simulink library "MESSIN_Library"  (R2024a)
settings: Solver=VariableStepAuto  StartTime=0.0  StopTime=10.0  RelTol=1e-3
undefined symbols (not defined in the file or in its folder): actuatorCommand, commandedActuator, commandMode, externCommand, ready, remoteControlDevice, sensor, supervisor, timestampUTC, useXNAllocation
libraries: $bdroot x376, etargetslib x52, simulink x19
(part 1 of 5)
settings Model: Creator=damerius  LastModifiedBy=Scythe
settings OptimizationCC: ReuseModelBlockBuffer=off
settings RTWCC: GPUComputeCapability=3.5

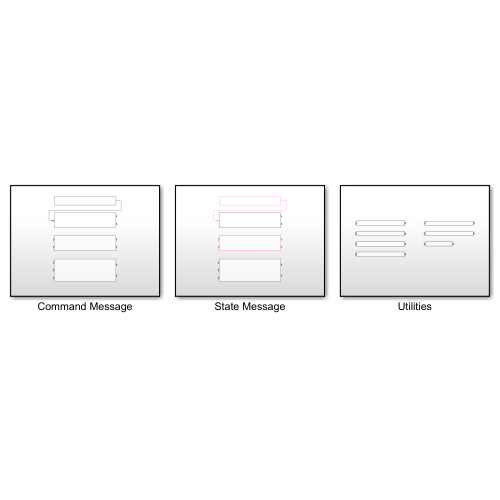
[thumbnail: Simulink's stored preview of the top-level diagram]
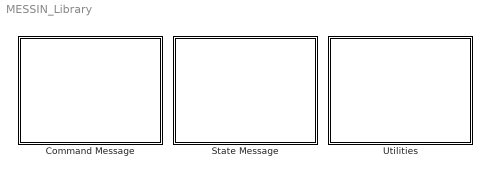
== system MESSIN_Library ==
  Command Message : Subsystem
  State Message : Subsystem
  Utilities : Subsystem

== system MESSIN_Library/Command Message ==
  Empty MESSIN Command Bus : Subsystem
      mask help: Construct an empty MESSIN command bus with default values.
      mask DialogControl DescGroupVar Prompt: Empty MESSIN Command Bus
      mask Display:
      | text(0.05, 0.5, '{\bfEmpty Bus}','horizontalAlignment','left','verticalAlignment','bottom','texmode','on');
      | text(0.05, 0.5, 'messinCommand','horizontalAlignment','left','verticalAlignment','top');
  Pack MESSIN Command Message : Subsystem
      mask help: Pack a MESSIN command message from the MESSIN command bus.
      mask DialogControl DescGroupVar Prompt: Pack MESSIN Command Message
      mask Display:
      | text(0.5, 0.5, '{\bfPack Message}','horizontalAlignment','center','verticalAlignment','bottom','texmode','on');
      | text(0.5, 0.5, 'MESSIN Command Message','horizontalAlignment','center','verticalAlignment','top');
  Unpack All MESSIN Command Messages : Subsystem
      mask help: Unpack all MESSIN command messages and construct a MESSIN command bus. If unpacking failed, then the success output returns false.
      mask DialogControl DescGroupVar Prompt: Unpack All MESSIN Command Messages
      mask Display:
      | text(0.5, 0.5, '{\bfUnpack All Messages}','horizontalAlignment','center','verticalAlignment','bottom','texmode','on');
      | text(0.5, 0.5, 'MESSIN Command Message','horizontalAlignment','center','verticalAlignment','top');
  Unpack MESSIN Command Message : Subsystem
      mask help: Unpack a MESSIN command message and construct a MESSIN command bus. If unpacking failed, then the success output returns false.
      mask DialogControl DescGroupVar Prompt: Unpack MESSIN Command Message
      mask Display:
      | text(0.5, 0.5, '{\bfUnpack Message}','horizontalAlignment','center','verticalAlignment','bottom','texmode','on');
      | text(0.5, 0.5, 'MESSIN Command Message','horizontalAlignment','center','verticalAlignment','top');
  wires:
  Empty MESSIN Command Bus/1(messinCommand) -> Pack MESSIN Command Message/1(messinCommand)

== system MESSIN_Library/State Message ==
  Empty MESSIN State Bus : Subsystem
      mask help: Construct an empty MESSIN state bus with default values.
      mask DialogControl DescGroupVar Prompt: Empty MESSIN State Bus
      mask Display:
      | text(0.05, 0.5, '{\bfEmpty Bus}','horizontalAlignment','left','verticalAlignment','bottom','texmode','on');
      | text(0.05, 0.5, 'messinState','horizontalAlignment','left','verticalAlignment','top');
  Pack MESSIN State Message : Subsystem
      mask help: Pack a MESSIN state message from the MESSIN state bus.
      mask DialogControl DescGroupVar Prompt: Pack MESSIN State Message
      mask Display:
      | text(0.5, 0.5, '{\bfPack Message}','horizontalAlignment','center','verticalAlignment','bottom','texmode','on');
      | text(0.5, 0.5, 'MESSIN State Message','horizontalAlignment','center','verticalAlignment','top');
  Unpack All MESSIN State Messages : Subsystem
      mask help: Unpack all MESSIN state messages and construct a MESSIN state bus. If unpacking failed, then the success output returns false.
      mask DialogControl DescGroupVar Prompt: Unpack All MESSIN State Messages
      mask Display:
      | text(0.5, 0.5, '{\bfUnpack All Messages}','horizontalAlignment','center','verticalAlignment','bottom','texmode','on');
      | text(0.5, 0.5, 'MESSIN State Message','horizontalAlignment','center','verticalAlignment','top');
  Unpack MESSIN State Message : Subsystem
      mask help: Unpack a MESSIN state message and construct a MESSIN state bus. If unpacking failed, then the success output returns false.
      mask DialogControl DescGroupVar Prompt: Unpack MESSIN State Message
      mask Display:
      | text(0.5, 0.5, '{\bfUnpack Message}','horizontalAlignment','center','verticalAlignment','bottom','texmode','on');
      | text(0.5, 0.5, 'MESSIN State Message','horizontalAlignment','center','verticalAlignment','top');
  wires:
  Empty MESSIN State Bus/1(messinState) -> Pack MESSIN State Message/1(messinState)

== system MESSIN_Library/Utilities ==
  Convert Double Network Byte Order : Subsystem
      mask DialogControl DescGroupVar Prompt: Convert Double Network Byte Order
      mask Display: disp('Network Byte Order (double)');
  Convert Single Network Byte Order : Subsystem
      mask DialogControl DescGroupVar Prompt: Convert Single Network Byte Order
      mask Display: disp('Network Byte Order (single)');
  Convert Uint16 Network Byte Order : Subsystem
      mask DialogControl DescGroupVar Prompt: Convert Uint16 Network Byte Order
      mask Display: disp('Network Byte Order (uint16)');
  Convert Uint32 Network Byte Order : Subsystem
      mask DialogControl DescGroupVar Prompt: Convert Uint32 Network Byte Order
      mask Display: disp('Network Byte Order (uint32)');
  Make Finite : Subsystem
      mask help: Make all values finite by replacing nonfinite values by zero.
      mask DialogControl DescGroupVar Prompt: Make Finite
      mask Display: disp('Make Finite');
  Pack Bitfield : Subsystem
      mask help: Convert a bitfield of 8 bits to a single byte. The input bitfield must be a vector containing 8 boolean values where the first value indicates whether the LSBit is to be set or not.
      mask DialogControl DescGroupVar Prompt: Pack Bitfield
      mask Display: disp('Pack Bitfield');
  Unpack Bitfield : Subsystem
      mask help: Extract all bits from a single byte. The bitfield output contains 8 boolean values where the first value indicates whether the LSBit is set or not.
      mask DialogControl DescGroupVar Prompt: Unpack Bitfield
      mask Display: disp('Unpack Bitfield');

== system MESSIN_Library/Command Message/Empty MESSIN Command Bus ==
  Bus Creator : BusCreator  Inputs=6
  Constant : Constant  Value=0.0  OutDataTypeStr=double
  Constant1 : Constant  Value=0  OutDataTypeStr=uint8
  Constant2 : Constant  Value=false  OutDataTypeStr=boolean
  Constant3 : Constant  Value=false  OutDataTypeStr=boolean
  Empty Actuator Command Bus : Subsystem
  Empty Allocation Command Bus : Subsystem
  Signal Specification : SignalSpecification  OutDataTypeStr=double  Unit=s  Dimensions=1
  Signal Specification1 : SignalSpecification  OutDataTypeStr=uint8  Dimensions=1
  Signal Specification2 : SignalSpecification  OutDataTypeStr=boolean  Dimensions=1
  Signal Specification3 : SignalSpecification  OutDataTypeStr=boolean  Dimensions=1
  messinCommand : Outport
  wires:
  Constant/1 -> Signal Specification/1
  Signal Specification/1 -> Bus Creator/1  "timestampUTC"
  Bus Creator/1 -> messinCommand/1
  Empty Actuator Command Bus/1(actuatorCommand) -> Bus Creator/5  "actuatorCommand"
  Empty Allocation Command Bus/1(allocationCommand) -> Bus Creator/6  "allocationCommand"
  Constant1/1 -> Signal Specification1/1
  Signal Specification1/1 -> Bus Creator/4  "commandMode"
  Constant2/1 -> Signal Specification2/1
  Signal Specification2/1 -> Bus Creator/2  "ready"
  Constant3/1 -> Signal Specification3/1
  Signal Specification3/1 -> Bus Creator/3  "useXNAllocation"

== system MESSIN_Library/Command Message/Pack MESSIN Command Message ==
  note: Info
  note: Commands
  note: Header
  messinCommand : Inport
  Bus Selector : BusSelector  OutputSignals=actuatorCommand
  Bus Selector1 : BusSelector  OutputSignals=allocationCommand
  Pack ActuatorCommand : Subsystem
  Pack AllocationCommand : Subsystem
  Pack Header : Subsystem
  Pack Info : Subsystem
  Vector Concatenate1 : Concatenate  NumInputs=4
  Width : Width  DataType=uint32
  messinCommand1 : InportShadow
  bytes : Outport  OutDataTypeStr=uint8
  length : Outport  Port=2  OutDataTypeStr=uint32  PortDimensions=1
  wires:
  messinCommand/1 -> Pack Info/1(messinCommand)
  Width/1 -> length/1
  Vector Concatenate1/1 -> Width/1, bytes/1
  messinCommand1/1 -> Bus Selector1/1, Bus Selector/1
  Bus Selector/1 -> Pack ActuatorCommand/1(actuatorCommand)  "<actuatorCommand>"
  Pack ActuatorCommand/1(bytes) -> Vector Concatenate1/3
  Pack Header/1(bytes) -> Vector Concatenate1/1
  Pack Info/1(bytes) -> Vector Concatenate1/2
  Bus Selector1/1 -> Pack AllocationCommand/1(allocationCommand)  "<allocationCommand>"
  Pack AllocationCommand/1(bytes) -> Vector Concatenate1/4

== system MESSIN_Library/Command Message/Unpack All MESSIN Command Messages ==
  note: protection for invalid input dimension
  bytes : Inport  OutDataTypeStr=uint8
  length : Inport  Port=2  OutDataTypeStr=uint32
  numMessages : Inport  Port=3  OutDataTypeStr=uint32  PortDimensions=1
  AND : Logic  Inputs=3  AllPortsSameDT=off  OutDataTypeStr=boolean
  Compare To Zero : simulink/Logic and Bit Operations/Compare To Zero  relop=>  OutDataTypeStr=boolean
  Compare To Zero1 : simulink/Logic and Bit Operations/Compare To Zero  relop=>  OutDataTypeStr=boolean
  Probe : Probe  ProbeWidth=off  ProbeSampleTime=off  ProbeComplexSignal=off  ProbeSignalDimensions=on  ProbeDimensionsDataType=uint32
  Relational Operator : RelationalOperator  Operator===  OutDataTypeStr=boolean  RndMeth=Simplest  InputSameDT=off
  Selector : Selector  InputPortWidth=2  IndexOptions=Index vector (dialog)  Indices=2  OutputSizes=1
  Sum of Elements : Sum  Inputs=+
  Width1 : Width  DataType=uint32
  run unpacking : Subsystem
  success : Outport  OutDataTypeStr=boolean  PortDimensions=1
  messinCommand : Outport  Port=2
  wires:
  run unpacking/1(messinCommand) -> messinCommand/1
  Compare To Zero1/1 -> AND/3
  run unpacking/2(vecUnpacked) -> Sum of Elements/1
  Relational Operator/1 -> AND/1, run unpacking/Enable
  Probe/1 -> Selector/1
  length/1 -> run unpacking/2(length), Width1/1
  Selector/1 -> Relational Operator/1
  bytes/1 -> Probe/1, run unpacking/1(bytes)
  numMessages/1 -> run unpacking/3(numMessages), Compare To Zero1/1
  AND/1 -> success/1
  Compare To Zero/1 -> AND/2
  Sum of Elements/1 -> Compare To Zero/1
  Width1/1 -> Relational Operator/2

== system MESSIN_Library/Command Message/Unpack MESSIN Command Message ==
  note: check length and header bytes
  bytes : Inport  OutDataTypeStr=uint8
  length : Inport  Port=2  OutDataTypeStr=uint32  PortDimensions=1
  is a valid message : Subsystem
  unpack message : Subsystem  TreatAsAtomicUnit=on
  success : Outport  OutDataTypeStr=boolean  PortDimensions=1
  messinCommand : Outport  Port=2
  wires:
  unpack message/1(messinCommand) -> messinCommand/1
  is a valid message/1(validMessage) -> success/1, unpack message/Enable
  length/1 -> is a valid message/1(length)
  bytes/1 -> is a valid message/2(bytes), unpack message/1(bytes)

== system MESSIN_Library/State Message/Empty MESSIN State Bus ==
  Bus Creator : BusCreator  Inputs=8
  Bus Creator1 : BusCreator  Inputs=6
  Bus Creator2 : BusCreator  Inputs=3
  Constant1 : Constant  Value=0.0  OutDataTypeStr=double
  Empty AirMAR Bus : Subsystem
  Empty BMS Bus : Subsystem
  Empty Commanded Actuator Bus : Subsystem
  Empty Control Bus : Subsystem
  Empty DVL Bus : Subsystem
  Empty GNSS Bus : Subsystem
  Empty Guidance Bus : Subsystem
  Empty INS Bus : Subsystem
  Empty MESSIN Command Bus : $bdroot/Command Message/Empty MESSIN Command Bus
  Empty MessinDrive Bus : Subsystem
  Empty Navigation Bus : Subsystem
  Empty RCD Bus : Subsystem
  Empty Supervisor Bus : Subsystem
  Empty System Diagnostics Bus : Subsystem
  Signal Specification : SignalSpecification  OutDataTypeStr=double  Unit=s  Dimensions=1
  messinState : Outport
  wires:
  Bus Creator/1 -> messinState/1
  Constant1/1 -> Signal Specification/1
  Bus Creator1/1 -> Bus Creator/2  "sensor"
  Empty RCD Bus/1(rcd) -> Bus Creator/3  "remoteControlDevice"
  Empty MessinDrive Bus/1(messinDrive) -> Bus Creator1/6  "messinDrive"
  Empty Control Bus/1(control) -> Bus Creator2/3  "control"
  Empty System Diagnostics Bus/1(systemDiagnostics) -> Bus Creator/7  "systemDiagnostics"
  Bus Creator2/1 -> Bus Creator/5  "gnc"
  Empty Supervisor Bus/1(supervisor) -> Bus Creator/4  "supervisor"
  Empty Guidance Bus/1(guidance) -> Bus Creator2/1  "guidance"
  Empty AirMAR Bus/1(airMAR) -> Bus Creator1/4  "airMAR"
  Empty Commanded Actuator Bus/1(commandedActuator) -> Bus Creator/6  "commandedActuator"
  Empty Navigation Bus/1(navigation) -> Bus Creator2/2  "navigation"
  Empty BMS Bus/1(batteryManagementSystem) -> Bus Creator1/5  "batteryManagementSystem"
  Empty DVL Bus/1(nortekDVL1000) -> Bus Creator1/3  "nortekDVL1000"
  Empty INS Bus/1(insLFK100) -> Bus Creator1/1  "insLFK100"
  Empty GNSS Bus/1(gnssAsteRx3) -> Bus Creator1/2  "gnssAsteRx3"
  Signal Specification/1 -> Bus Creator/1  "timestampUTC"
  Empty MESSIN Command Bus/1 -> Bus Creator/8  "externCommand"

== system MESSIN_Library/State Message/Pack MESSIN State Message ==
  note: Sensor
  note: Header
  note: Info
  note: RCD
  note: Supervisor
  note: GNC
  note: System Diagnostics
  note: Extern Command
  messinState : Inport
  Bus Selector : BusSelector  OutputSignals=sensor
  Bus Selector1 : BusSelector  OutputSignals=nortekDVL1000
  Bus Selector10 : BusSelector  OutputSignals=externCommand
  Bus Selector18 : BusSelector  OutputSignals=messinDrive
  Bus Selector19 : BusSelector  OutputSignals=remoteControlDevice
  Bus Selector2 : BusSelector  OutputSignals=insLFK100
  Bus Selector3 : BusSelector  OutputSignals=supervisor
  Bus Selector4 : BusSelector  OutputSignals=batteryManagementSystem
  Bus Selector5 : BusSelector  OutputSignals=gnc
  Bus Selector6 : BusSelector  OutputSignals=airMAR
  Bus Selector7 : BusSelector  OutputSignals=gnssAsteRx3
  Bus Selector8 : BusSelector  OutputSignals=commandedActuator
  Bus Selector9 : BusSelector  OutputSignals=systemDiagnostics
  Pack AirMAR : Subsystem
  Pack BMS : Subsystem
  Pack CommandedActuator : Subsystem
  Pack DVL : Subsystem
  Pack ExternCommand : Subsystem
  Pack GNC : Subsystem
  Pack GNSS : Subsystem
  Pack Header : Subsystem
  Pack INS : Subsystem
  Pack Info : Subsystem
  Pack MessinDrive : Subsystem
  Pack RCD : Subsystem
  Pack Supervisor : Subsystem
  Pack SystemDiagnostics : Subsystem
  Vector Concatenate1 : Concatenate  NumInputs=9
  Vector Concatenate2 : Concatenate  NumInputs=6
  Width : Width  DataType=uint32
  bytes : Outport  OutDataTypeStr=uint8
  length : Outport  Port=2  OutDataTypeStr=uint32  PortDimensions=1
  wires:
  Width/1 -> length/1
  Vector Concatenate1/1 -> bytes/1, Width/1
  Bus Selector2/1 -> Pack INS/1(insLFK100)  "<insLFK100>"
  Bus Selector/1 -> Bus Selector18/1, Bus Selector4/1, Bus Selector6/1, Bus Selector1/1, Bus Selector7/1, Bus Selector2/1  "<sensor>"
  messinState/1 -> Bus Selector10/1, Bus Selector9/1, Bus Selector8/1, Bus Selector5/1, Bus Selector3/1, Bus Selector19/1, Bus Selector/1, Pack Info/1(messinState)
  Bus Selector1/1 -> Pack DVL/1(dvl)  "<nortekDVL1000>"
  Bus Selector4/1 -> Pack BMS/1(bms)  "<batteryManagementSystem>"
  Bus Selector6/1 -> Pack AirMAR/1(airMAR)  "<airMAR>"
  Bus Selector7/1 -> Pack GNSS/1(gnss)  "<gnssAsteRx3>"
  Pack DVL/1(bytes) -> Vector Concatenate2/3
  Pack AirMAR/1(bytes) -> Vector Concatenate2/4
  Pack GNSS/1(bytes) -> Vector Concatenate2/2
  Pack BMS/1(bytes) -> Vector Concatenate2/5
  Pack INS/1(bytes) -> Vector Concatenate2/1
  Pack Header/1(bytes) -> Vector Concatenate1/1
  Pack Info/1(bytes) -> Vector Concatenate1/2
  Vector Concatenate2/1 -> Vector Concatenate1/3
  Bus Selector18/1 -> Pack MessinDrive/1(messinDrive)  "<messinDrive>"
  Pack MessinDrive/1(bytes) -> Vector Concatenate2/6
  Bus Selector19/1 -> Pack RCD/1(rcd)  "<remoteControlDevice>"
  Pack RCD/1(bytes) -> Vector Concatenate1/4
  Bus Selector3/1 -> Pack Supervisor/1(supervisor)  "<supervisor>"
  Pack Supervisor/1(bytes) -> Vector Concatenate1/5
  Bus Selector5/1 -> Pack GNC/1(gnc)  "<gnc>"
  Pack GNC/1(bytes) -> Vector Concatenate1/6
  Bus Selector8/1 -> Pack CommandedActuator/1(commandedActuator)  "<commandedActuator>"
  Pack CommandedActuator/1(bytes) -> Vector Concatenate1/7
  Bus Selector9/1 -> Pack SystemDiagnostics/1(systemDiagnostics)  "<systemDiagnostics>"
  Pack SystemDiagnostics/1(bytes) -> Vector Concatenate1/8
  Bus Selector10/1 -> Pack ExternCommand/1(externCommand)  "<externCommand>"
  Pack ExternCommand/1(bytes) -> Vector Concatenate1/9

== system MESSIN_Library/State Message/Unpack All MESSIN State Messages ==
  note: protection for invalid input dimension
  bytes : Inport  OutDataTypeStr=uint8
  length : Inport  Port=2  OutDataTypeStr=uint32
  numMessages : Inport  Port=3  OutDataTypeStr=uint32  PortDimensions=1
  AND : Logic  Inputs=3  AllPortsSameDT=off  OutDataTypeStr=boolean
  Compare To Zero : simulink/Logic and Bit Operations/Compare To Zero  relop=>  OutDataTypeStr=boolean
  Compare To Zero1 : simulink/Logic and Bit Operations/Compare To Zero  relop=>  OutDataTypeStr=boolean
  Probe : Probe  ProbeWidth=off  ProbeSampleTime=off  ProbeComplexSignal=off  ProbeSignalDimensions=on  ProbeDimensionsDataType=uint32
  Relational Operator : RelationalOperator  Operator===  OutDataTypeStr=boolean  RndMeth=Simplest  InputSameDT=off
  Selector : Selector  InputPortWidth=2  IndexOptions=Index vector (dialog)  Indices=2  OutputSizes=1
  Sum of Elements : Sum  Inputs=+
  Width1 : Width  DataType=uint32
  run unpacking : Subsystem
  success : Outport  OutDataTypeStr=boolean  PortDimensions=1
  messinState : Outport  Port=2
  wires:
  Selector/1 -> Relational Operator/1
  bytes/1 -> Probe/1, run unpacking/1(bytes)
  Sum of Elements/1 -> Compare To Zero/1
  Width1/1 -> Relational Operator/2
  Probe/1 -> Selector/1
  Compare To Zero/1 -> AND/2
  length/1 -> run unpacking/2(length), Width1/1
  AND/1 -> success/1
  run unpacking/2(vecUnpacked) -> Sum of Elements/1
  Relational Operator/1 -> AND/1, run unpacking/Enable
  numMessages/1 -> run unpacking/3(numMessages), Compare To Zero1/1
  run unpacking/1(messinState) -> messinState/1
  Compare To Zero1/1 -> AND/3

== system MESSIN_Library/State Message/Unpack MESSIN State Message ==
  note: check length and header bytes
  bytes : Inport  OutDataTypeStr=uint8
  length : Inport  Port=2  OutDataTypeStr=uint32  PortDimensions=1
  is a valid message : Subsystem
  unpack message : Subsystem  TreatAsAtomicUnit=on
  success : Outport  OutDataTypeStr=boolean  PortDimensions=1
  messinState : Outport  Port=2
  wires:
  is a valid message/1(validMessage) -> success/1, unpack message/Enable
  bytes/1 -> is a valid message/2(bytes), unpack message/1(bytes)
  unpack message/1(messinState) -> messinState/1
  length/1 -> is a valid message/1(length)

== system MESSIN_Library/Utilities/Convert Double Network Byte Order ==
  note: Check endianess of this machine
      | (only swap on little-endian-based machines)
  in : Inport  OutDataTypeStr=double  PortDimensions=1
  Byte Pack : etargetslib/Byte Pack  datatypes={'double'}  byteAlign=1
  Byte Pack1 : etargetslib/Byte Pack  datatypes={'uint16'}  byteAlign=1
  Byte Unpack : etargetslib/Byte Unpack  dimensions={[1]}  datatypes={'double'}  byteAlign=1
  Constant : Constant  Value=uint16(1)
  Selector : Selector  InputPortWidth=8  IndexOptions=Index vector (dialog)  Indices=[8 7 6 5 4 3 2 1]  OutputSizes=1
  Selector2 : Selector  InputPortWidth=2  IndexOptions=Index vector (dialog)  Indices=1  OutputSizes=1
  Switch : Switch  Criteria=u2 ~= 0  SaturateOnIntegerOverflow=off  InputSameDT=off
  out : Outport  OutDataTypeStr=double  PortDimensions=1
  wires:
  Byte Unpack/1 -> Switch/1
  Selector/1 -> Byte Unpack/1
  Constant/1 -> Byte Pack1/1
  in/1 -> Switch/3, Byte Pack/1
  Selector2/1 -> Switch/2
  Byte Pack/1 -> Selector/1
  Byte Pack1/1 -> Selector2/1
  Switch/1 -> out/1

== system MESSIN_Library/Utilities/Convert Single Network Byte Order ==
  note: Check endianess of this machine
      | (only swap on little-endian-based machines)
  in : Inport  OutDataTypeStr=single  PortDimensions=1
  Byte Pack : etargetslib/Byte Pack  datatypes={'single'}  byteAlign=1
  Byte Pack1 : etargetslib/Byte Pack  datatypes={'uint16'}  byteAlign=1
  Byte Unpack : etargetslib/Byte Unpack  dimensions={[1]}  datatypes={'single'}  byteAlign=1
  Constant : Constant  Value=uint16(1)
  Selector : Selector  InputPortWidth=4  IndexOptions=Index vector (dialog)  Indices=[4 3 2 1]  OutputSizes=1
  Selector2 : Selector  InputPortWidth=2  IndexOptions=Index vector (dialog)  Indices=1  OutputSizes=1
  Switch : Switch  Criteria=u2 ~= 0  SaturateOnIntegerOverflow=off  InputSameDT=off
  out : Outport  OutDataTypeStr=single  PortDimensions=1
  wires:
  Switch/1 -> out/1
  Byte Pack1/1 -> Selector2/1
  Byte Pack/1 -> Selector/1
  Selector2/1 -> Switch/2
  in/1 -> Byte Pack/1, Switch/3
  Constant/1 -> Byte Pack1/1
  Selector/1 -> Byte Unpack/1
  Byte Unpack/1 -> Switch/1

== system MESSIN_Library/Utilities/Convert Uint16 Network Byte Order ==
  note: Check endianess of this machine
      | (only swap on little-endian-based machines)
  in : Inport  OutDataTypeStr=uint16  PortDimensions=1
  Byte Pack : etargetslib/Byte Pack  datatypes={'uint16'}  byteAlign=1
  Byte Pack1 : etargetslib/Byte Pack  datatypes={'uint16'}  byteAlign=1
  Byte Unpack : etargetslib/Byte Unpack  dimensions={[1]}  datatypes={'uint16'}  byteAlign=1
  Constant : Constant  Value=uint16(1)
  Selector : Selector  InputPortWidth=2  IndexOptions=Index vector (dialog)  Indices=[2 1]  OutputSizes=1
  Selector2 : Selector  InputPortWidth=2  IndexOptions=Index vector (dialog)  Indices=1  OutputSizes=1
  Switch : Switch  Criteria=u2 ~= 0  SaturateOnIntegerOverflow=off  InputSameDT=off
  out : Outport  OutDataTypeStr=uint16  PortDimensions=1
  wires:
  Byte Unpack/1 -> Switch/1
  Selector/1 -> Byte Unpack/1
  Constant/1 -> Byte Pack1/1
  in/1 -> Switch/3, Byte Pack/1
  Selector2/1 -> Switch/2
  Byte Pack/1 -> Selector/1
  Byte Pack1/1 -> Selector2/1
  Switch/1 -> out/1

== system MESSIN_Library/Utilities/Convert Uint32 Network Byte Order ==
  note: Check endianess of this machine
      | (only swap on little-endian-based machines)
  in : Inport  OutDataTypeStr=uint32  PortDimensions=1
  Byte Pack : etargetslib/Byte Pack  datatypes={'uint32'}  byteAlign=1
  Byte Pack1 : etargetslib/Byte Pack  datatypes={'uint16'}  byteAlign=1
  Byte Unpack : etargetslib/Byte Unpack  dimensions={[1]}  datatypes={'uint32'}  byteAlign=1
  Constant : Constant  Value=uint16(1)
  Selector : Selector  InputPortWidth=4  IndexOptions=Index vector (dialog)  Indices=[4 3 2 1]  OutputSizes=1
  Selector2 : Selector  InputPortWidth=2  IndexOptions=Index vector (dialog)  Indices=1  OutputSizes=1
  Switch : Switch  Criteria=u2 ~= 0  SaturateOnIntegerOverflow=off  InputSameDT=off
  out : Outport  OutDataTypeStr=uint32  PortDimensions=1
  wires:
  Switch/1 -> out/1
  Byte Pack1/1 -> Selector2/1
  Byte Pack/1 -> Selector/1
  Selector2/1 -> Switch/2
  in/1 -> Byte Pack/1, Switch/3
  Constant/1 -> Byte Pack1/1
  Selector/1 -> Byte Unpack/1
  Byte Unpack/1 -> Switch/1

== system MESSIN_Library/Utilities/Make Finite ==
  in : Inport  OutDataTypeStr=double
  ReplaceNonfiniteByZeros : MATLAB Function  TreatAsAtomicUnit=on
  out : Outport  OutDataTypeStr=double
  wires:
  in/1 -> ReplaceNonfiniteByZeros/1(u)
  ReplaceNonfiniteByZeros/1(y) -> out/1

== system MESSIN_Library/Utilities/Pack Bitfield ==
  bitfield : Inport  OutDataTypeStr=boolean  PortDimensions=8
  Bitwise Operator : simulink/Logic and Bit Operations/Bitwise Operator  logicop=OR  UseBitMask=off  NumInputPorts=8  BitMask=bin2dec('11011001')  BitMaskRealWorld=Stored Integer
  Data Type Conversion : DataTypeConversion  OutDataTypeStr=uint8  SaturateOnIntegerOverflow=off  RndMeth=Floor
  Demux : Demux  Outputs=8
  Shift Arithmetic : ArithShift  BitShiftNumber=1  BitShiftDirection=Left
  Shift Arithmetic1 : ArithShift  BitShiftNumber=2  BitShiftDirection=Left
  Shift Arithmetic2 : ArithShift  BitShiftNumber=3  BitShiftDirection=Left
  Shift Arithmetic3 : ArithShift  BitShiftNumber=4  BitShiftDirection=Left
  Shift Arithmetic4 : ArithShift  BitShiftNumber=5  BitShiftDirection=Left
  Shift Arithmetic5 : ArithShift  BitShiftNumber=6  BitShiftDirection=Left
  Shift Arithmetic6 : ArithShift  BitShiftNumber=7  BitShiftDirection=Left
  byte : Outport  OutDataTypeStr=uint8  PortDimensions=1
  wires:
  Demux/8 -> Shift Arithmetic6/1
  Shift Arithmetic2/1 -> Bitwise Operator/4
  Shift Arithmetic5/1 -> Bitwise Operator/7
  Shift Arithmetic6/1 -> Bitwise Operator/8
  Shift Arithmetic4/1 -> Bitwise Operator/6
  Data Type Conversion/1 -> Demux/1
  Shift Arithmetic/1 -> Bitwise Operator/2
  Shift Arithmetic3/1 -> Bitwise Operator/5
  Demux/2 -> Shift Arithmetic/1
  Demux/7 -> Shift Arithmetic5/1
  Demux/5 -> Shift Arithmetic3/1
  Demux/4 -> Shift Arithmetic2/1
  Demux/6 -> Shift Arithmetic4/1
  Demux/3 -> Shift Arithmetic1/1
  Shift Arithmetic1/1 -> Bitwise Operator/3
  Demux/1 -> Bitwise Operator/1
  bitfield/1 -> Data Type Conversion/1
  Bitwise Operator/1 -> byte/1

== system MESSIN_Library/Utilities/Unpack Bitfield ==
  byte : Inport  OutDataTypeStr=uint8  PortDimensions=1
  Bitwise Operator : simulink/Logic and Bit Operations/Bitwise Operator  logicop=AND  UseBitMask=on  BitMask=1  BitMaskRealWorld=Stored Integer
  Bitwise Operator1 : simulink/Logic and Bit Operations/Bitwise Operator  logicop=AND  UseBitMask=on  BitMask=2  BitMaskRealWorld=Stored Integer
  Bitwise Operator2 : simulink/Logic and Bit Operations/Bitwise Operator  logicop=AND  UseBitMask=on  BitMask=4  BitMaskRealWorld=Stored Integer
  Bitwise Operator3 : simulink/Logic and Bit Operations/Bitwise Operator  logicop=AND  UseBitMask=on  BitMask=8  BitMaskRealWorld=Stored Integer
  Bitwise Operator4 : simulink/Logic and Bit Operations/Bitwise Operator  logicop=AND  UseBitMask=on  BitMask=16  BitMaskRealWorld=Stored Integer
  Bitwise Operator5 : simulink/Logic and Bit Operations/Bitwise Operator  logicop=AND  UseBitMask=on  BitMask=32  BitMaskRealWorld=Stored Integer
  Bitwise Operator6 : simulink/Logic and Bit Operations/Bitwise Operator  logicop=AND  UseBitMask=on  BitMask=64  BitMaskRealWorld=Stored Integer
  Bitwise Operator7 : simulink/Logic and Bit Operations/Bitwise Operator  logicop=AND  UseBitMask=on  BitMask=128  BitMaskRealWorld=Stored Integer
  Data Type Conversion1 : DataTypeConversion  OutDataTypeStr=boolean  SaturateOnIntegerOverflow=off  RndMeth=Floor
  Mux : Mux  Inputs=8
  bitfield : Outport  OutDataTypeStr=boolean  PortDimensions=8
  wires:
  Mux/1 -> Data Type Conversion1/1
  Bitwise Operator1/1 -> Mux/2
  byte/1 -> Bitwise Operator/1, Bitwise Operator7/1, Bitwise Operator6/1, Bitwise Operator5/1, Bitwise Operator4/1, Bitwise Operator3/1, Bitwise Operator2/1, Bitwise Operator1/1
  Bitwise Operator/1 -> Mux/1
  Bitwise Operator4/1 -> Mux/5
  Bitwise Operator3/1 -> Mux/4
  Bitwise Operator2/1 -> Mux/3
  Bitwise Operator5/1 -> Mux/6
  Bitwise Operator7/1 -> Mux/8
  Bitwise Operator6/1 -> Mux/7
  Data Type Conversion1/1 -> bitfield/1

== system MESSIN_Library/Command Message/Empty MESSIN Command Bus/Empty Actuator Command Bus ==
  Bus Creator6 : BusCreator  Inputs=4
  Constant{6..8,19} (4 alike) : Constant  Value=0.0  OutDataTypeStr=double
  Signal Specification18 : SignalSpecification  OutDataTypeStr=double  Unit=1  Dimensions=1
  Signal Specification6 : SignalSpecification  OutDataTypeStr=double  Unit=1  Dimensions=1
  Signal Specification7 : SignalSpecification  OutDataTypeStr=double  Unit=rad  Dimensions=1
  Signal Specification8 : SignalSpecification  OutDataTypeStr=double  Unit=rad  Dimensions=1
  actuatorCommand : Outport
  wires:
  Signal Specification8/1 -> Bus Creator6/4  "anglePortside"
  Bus Creator6/1 -> actuatorCommand/1
  Signal Specification18/1 -> Bus Creator6/1  "throttleStarboard"
  Constant6/1 -> Signal Specification6/1
  Constant8/1 -> Signal Specification8/1
  Signal Specification6/1 -> Bus Creator6/2  "throttlePortside"
  Signal Specification7/1 -> Bus Creator6/3  "angleStarboard"
  Constant7/1 -> Signal Specification7/1
  Constant19/1 -> Signal Specification18/1

== system MESSIN_Library/Command Message/Empty MESSIN Command Bus/Empty Allocation Command Bus ==
  Bus Creator : BusCreator  Inputs=1
  Constant1 : Constant  Value=[0;0;0]  OutDataTypeStr=double
  Signal Specification1 : SignalSpecification  OutDataTypeStr=double  Dimensions=3
  allocationCommand : Outport
  wires:
  Constant1/1 -> Signal Specification1/1
  Signal Specification1/1 -> Bus Creator/1  "XYN"
  Bus Creator/1 -> allocationCommand/1

== system MESSIN_Library/Command Message/Pack MESSIN Command Message/Pack ActuatorCommand ==
  actuatorCommand : Inport
  Bus Selector1 : BusSelector  OutputSignals=throttleStarboard,throttlePortside,angleStarboard,anglePortside
  Byte Pack : etargetslib/Byte Pack  datatypes={'double','double','double','double'}  byteAlign=1
  Convert Double Network Byte Order{,1..3} (4 alike) : $bdroot/Utilities/Convert Double Network Byte Order
  Data Type Conversion{,1..3} (4 alike) : DataTypeConversion  OutDataTypeStr=double  SaturateOnIntegerOverflow=off  RndMeth=Floor
  bytes : Outport
  wires:
  actuatorCommand/1 -> Bus Selector1/1
  Data Type Conversion3/1 -> Convert Double Network Byte Order3/1
  Data Type Conversion2/1 -> Convert Double Network Byte Order2/1
  Data Type Conversion1/1 -> Convert Double Network Byte Order1/1
  Data Type Conversion/1 -> Convert Double Network Byte Order/1
  Byte Pack/1 -> bytes/1
  Convert Double Network Byte Order/1 -> Byte Pack/1
  Convert Double Network Byte Order1/1 -> Byte Pack/2
  Convert Double Network Byte Order2/1 -> Byte Pack/3
  Convert Double Network Byte Order3/1 -> Byte Pack/4
  Bus Selector1/1 -> Data Type Conversion/1  "<throttleStarboard>"
  Bus Selector1/2 -> Data Type Conversion1/1  "<throttlePortside>"
  Bus Selector1/3 -> Data Type Conversion2/1  "<angleStarboard>"
  Bus Selector1/4 -> Data Type Conversion3/1  "<anglePortside>"

== system MESSIN_Library/Command Message/Pack MESSIN Command Message/Pack AllocationCommand ==
  allocationCommand : Inport
  Bus Selector1 : BusSelector  OutputSignals=XYN
  Byte Pack : etargetslib/Byte Pack  datatypes={'double','double','double'}  byteAlign=1
  Convert Double Network Byte Order : $bdroot/Utilities/Convert Double Network Byte Order
  Convert Double Network Byte Order1 : $bdroot/Utilities/Convert Double Network Byte Order
  Convert Double Network Byte Order2 : $bdroot/Utilities/Convert Double Network Byte Order
  Data Type Conversion : DataTypeConversion  OutDataTypeStr=double  SaturateOnIntegerOverflow=off  RndMeth=Floor
  Data Type Conversion1 : DataTypeConversion  OutDataTypeStr=double  SaturateOnIntegerOverflow=off  RndMeth=Floor
  Data Type Conversion2 : DataTypeConversion  OutDataTypeStr=double  SaturateOnIntegerOverflow=off  RndMeth=Floor
  Demux : Demux  Outputs=3
  bytes : Outport
  wires:
  Convert Double Network Byte Order2/1 -> Byte Pack/3
  Convert Double Network Byte Order1/1 -> Byte Pack/2
  Convert Double Network Byte Order/1 -> Byte Pack/1
  Byte Pack/1 -> bytes/1
  Data Type Conversion/1 -> Convert Double Network Byte Order/1
  Data Type Conversion1/1 -> Convert Double Network Byte Order1/1
  Data Type Conversion2/1 -> Convert Double Network Byte Order2/1
  allocationCommand/1 -> Bus Selector1/1
  Bus Selector1/1 -> Demux/1  "<XYN>"
  Demux/1 -> Data Type Conversion/1
  Demux/2 -> Data Type Conversion1/1
  Demux/3 -> Data Type Conversion2/1

== system MESSIN_Library/Command Message/Pack MESSIN Command Message/Pack Header ==
  note: M essin C ommand
  ID : Constant  Value=uint8('MC')  OutDataTypeStr=uint8
  bytes : Outport
  wires:
  ID/1 -> bytes/1

== system MESSIN_Library/Command Message/Pack MESSIN Command Message/Pack Info ==
  messinCommand : Inport
  Bus Selector1 : BusSelector  OutputSignals=timestampUTC
  Bus Selector2 : BusSelector  OutputSignals=ready,useXNAllocation
  Bus Selector3 : BusSelector  OutputSignals=commandMode
  Byte Pack : etargetslib/Byte Pack  datatypes={'double'}  byteAlign=1
  Cast To Boolean : DataTypeConversion  OutDataTypeStr=boolean  SaturateOnIntegerOverflow=off  RndMeth=Floor
  Cast To Boolean1 : DataTypeConversion  OutDataTypeStr=boolean  SaturateOnIntegerOverflow=off  RndMeth=Floor
  Constant : Constant  Value=false  OutDataTypeStr=boolean
  Convert Double Network Byte Order : $bdroot/Utilities/Convert Double Network Byte Order
  Data Type Conversion : DataTypeConversion  OutDataTypeStr=uint8  SaturateOnIntegerOverflow=off  RndMeth=Floor
  Mux : Mux  Inputs=8
  Pack Bitfield : $bdroot/Utilities/Pack Bitfield
  Selector : Selector  InputPortWidth=8  IndexOptions=Index vector (dialog)  Indices=[8 7 6 5 4 3 2 1]  OutputSizes=1
  Vector Concatenate : Concatenate  NumInputs=3
  bytes : Outport
  wires:
  Byte Pack/1 -> Vector Concatenate/1
  messinCommand/1 -> Bus Selector3/1, Bus Selector2/1, Bus Selector1/1
  Convert Double Network Byte Order/1 -> Byte Pack/1
  Bus Selector1/1 -> Convert Double Network Byte Order/1  "<timestampUTC>"
  Cast To Boolean/1 -> Mux/1
  Constant/1 -> Mux/7, Mux/6, Mux/5, Mux/4, Mux/3, Mux/8
  Mux/1 -> Selector/1
  Selector/1 -> Pack Bitfield/1
  Bus Selector2/1 -> Cast To Boolean/1  "<ready>"
  Bus Selector3/1 -> Data Type Conversion/1  "<commandMode>"
  Pack Bitfield/1 -> Vector Concatenate/2
  Data Type Conversion/1 -> Vector Concatenate/3
  Vector Concatenate/1 -> bytes/1
  Cast To Boolean1/1 -> Mux/2
  Bus Selector2/2 -> Cast To Boolean1/1  "<useXNAllocation>"

== system MESSIN_Library/Command Message/Unpack All MESSIN Command Messages/run unpacking ==
  bytes : Inport
  length : Inport  Port=2
  numMessages : Inport  Port=3
  Enable : EnablePort
  Gain : Gain  Gain=0  OutDataTypeStr=uint32
  unpack all in a loop : Subsystem  TreatAsAtomicUnit=on
  messinCommand : Outport
  vecUnpacked : Outport  Port=2
  wires:
  bytes/1 -> unpack all in a loop/1(bytes)
  unpack all in a loop/1(messinCommand) -> messinCommand/1
  unpack all in a loop/2(vecUnpacked) -> vecUnpacked/1
  length/1 -> unpack all in a loop/2(length), Gain/1
  Gain/1 -> unpack all in a loop/4(zeros)
  numMessages/1 -> unpack all in a loop/3(numMessages)

== system MESSIN_Library/Command Message/Unpack MESSIN Command Message/is a valid message ==
  length : Inport
  bytes : Inport  Port=2
  AND1 : Logic  AllPortsSameDT=off  OutDataTypeStr=boolean
  CheckHeaderBytes : Subsystem  TreatAsAtomicUnit=on
  CheckMessageLength : simulink/Logic and Bit Operations/Compare To Constant  relop===  const=uint32(68)  OutDataTypeStr=boolean
  Min : MinMax  Inputs=2
  Width : Width  DataType=uint32
  validMessage : Outport
  wires:
  CheckMessageLength/1 -> AND1/1, CheckHeaderBytes/Enable
  AND1/1 -> validMessage/1
  CheckHeaderBytes/1(validHeader) -> AND1/2
  length/1 -> Min/1
  Width/1 -> Min/2
  bytes/1 -> CheckHeaderBytes/1(bytes), Width/1
  Min/1 -> CheckMessageLength/1

== system MESSIN_Library/Command Message/Unpack MESSIN Command Message/unpack message ==
  note: Actuator Command
  note: Info
  note: Allocation Command
  bytes : Inport
  Enable : EnablePort
  Bytes 12 to 43 : Selector  IndexMode=Zero-based  IndexOptions=Index vector (dialog)  Indices=12:43  OutputSizes=1
  Bytes 2 to 11 : Selector  IndexMode=Zero-based  IndexOptions=Index vector (dialog)  Indices=2:11  OutputSizes=1
  Bytes 44 to 67 : Selector  IndexMode=Zero-based  IndexOptions=Index vector (dialog)  Indices=44:67  OutputSizes=1
  Empty MESSIN Command Bus : $bdroot/Command Message/Empty MESSIN Command Bus
  Unpack ActuatorCommand : Subsystem
  Unpack AllocationCommand : Subsystem
  Unpack Info : Subsystem
  messinCommand : Outport
  wires:
  Unpack Info/1(busOut) -> Unpack ActuatorCommand/1(busIn)
  Bytes 12 to 43/1 -> Unpack ActuatorCommand/2(bytes)
  Bytes 2 to 11/1 -> Unpack Info/2(bytes)
  Empty MESSIN Command Bus/1 -> Unpack Info/1(busIn)
  bytes/1 -> Bytes 2 to 11/1, Bytes 44 to 67/1, Bytes 12 to 43/1
  Bytes 44 to 67/1 -> Unpack AllocationCommand/2(bytes)
  Unpack AllocationCommand/1(busOut) -> messinCommand/1
  Unpack ActuatorCommand/1(busOut) -> Unpack AllocationCommand/1(busIn)

== system MESSIN_Library/State Message/Empty MESSIN State Bus/Empty AirMAR Bus ==
  Bus Creator2 : BusCreator  Inputs=3
  Bus Creator4 : BusCreator  Inputs=3
  Bus Creator5 : BusCreator  Inputs=2
  Constant{2..7} (6 alike) : Constant  Value=0.0  OutDataTypeStr=double
  Signal Specification1 : SignalSpecification  OutDataTypeStr=double  Unit=s  Dimensions=1
  Signal Specification2 : SignalSpecification  OutDataTypeStr=double  Unit=Pa  Dimensions=1
  Signal Specification3 : SignalSpecification  OutDataTypeStr=double  Unit=°C  Dimensions=1
  Signal Specification4 : SignalSpecification  OutDataTypeStr=double  Unit=s  Dimensions=1
  Signal Specification5 : SignalSpecification  OutDataTypeStr=double  Unit=rad  Dimensions=1
  Signal Specification6 : SignalSpecification  OutDataTypeStr=double  Unit=m/s  Dimensions=1
  airMAR : Outport
  wires:
  Signal Specification4/1 -> Bus Creator4/1  "timestampUTC"
  Constant2/1 -> Signal Specification1/1
  Constant5/1 -> Signal Specification4/1
  Signal Specification6/1 -> Bus Creator4/3  "windSpeed"
  Constant4/1 -> Signal Specification3/1
  Bus Creator5/1 -> airMAR/1
  Constant3/1 -> Signal Specification2/1
  Bus Creator2/1 -> Bus Creator5/1  "air"
  Signal Specification1/1 -> Bus Creator2/1  "timestampUTC"
  Signal Specification2/1 -> Bus Creator2/2  "pressure"
  Bus Creator4/1 -> Bus Creator5/2  "relativeWind"
  Signal Specification3/1 -> Bus Creator2/3  "airTemperature"
  Constant7/1 -> Signal Specification6/1
  Constant6/1 -> Signal Specification5/1
  Signal Specification5/1 -> Bus Creator4/2  "windAngle"

== system MESSIN_Library/State Message/Empty MESSIN State Bus/Empty BMS Bus ==
  Bus Creator3 : BusCreator  Inputs=5
  Bus Creator6 : BusCreator  Inputs=2
  Bus Creator7 : BusCreator  Inputs=5
  Constant{8..17} (10 alike) : Constant  Value=0.0  OutDataTypeStr=double
  Signal Specification10 : SignalSpecification  OutDataTypeStr=double  Unit=A*s  Dimensions=1
  Signal Specification11 : SignalSpecification  OutDataTypeStr=double  Unit=1  Dimensions=1
  Signal Specification12 : SignalSpecification  OutDataTypeStr=double  Unit=A*s  Dimensions=1
  Signal Specification13 : SignalSpecification  OutDataTypeStr=double  Unit=1  Dimensions=1
  Signal Specification14 : SignalSpecification  OutDataTypeStr=double  Unit=s  Dimensions=1
  Signal Specification15 : SignalSpecification  OutDataTypeStr=double  Unit=V  Dimensions=1
  Signal Specification16 : SignalSpecification  OutDataTypeStr=double  Unit=A  Dimensions=1
  Signal Specification7 : SignalSpecification  OutDataTypeStr=double  Unit=s  Dimensions=1
  Signal Specification8 : SignalSpecification  OutDataTypeStr=double  Unit=V  Dimensions=1
  Signal Specification9 : SignalSpecification  OutDataTypeStr=double  Unit=A  Dimensions=1
  batteryManagementSystem : Outport
  wires:
  Constant16/1 -> Signal Specification14/1
  Constant8/1 -> Signal Specification7/1
  Bus Creator6/1 -> batteryManagementSystem/1
  Constant9/1 -> Signal Specification8/1
  Constant13/1 -> Signal Specification16/1
  Constant15/1 -> Signal Specification13/1
  Signal Specification9/1 -> Bus Creator3/3  "current"
  Bus Creator7/1 -> Bus Creator6/2  "batteryPortside"
  Signal Specification15/1 -> Bus Creator7/2  "voltage"
  Signal Specification13/1 -> Bus Creator7/5  "stateOfCharge"
  Signal Specification7/1 -> Bus Creator3/1  "timestampUTC"
  Constant17/1 -> Signal Specification15/1
  Constant12/1 -> Signal Specification11/1
  Signal Specification12/1 -> Bus Creator7/4  "consumedElectricCharge"
  Signal Specification14/1 -> Bus Creator7/1  "timestampUTC"
  Signal Specification8/1 -> Bus Creator3/2  "voltage"
  Signal Specification16/1 -> Bus Creator7/3  "current"
  Constant11/1 -> Signal Specification10/1
  Bus Creator3/1 -> Bus Creator6/1  "batteryStarboard"
  Signal Specification11/1 -> Bus Creator3/5  "stateOfCharge"
  Constant10/1 -> Signal Specification9/1
  Constant14/1 -> Signal Specification12/1
  Signal Specification10/1 -> Bus Creator3/4  "consumedElectricCharge"

== system MESSIN_Library/State Message/Empty MESSIN State Bus/Empty Commanded Actuator Bus ==
  Bus Creator6 : BusCreator  Inputs=4
  Constant{1..3,19} (4 alike) : Constant  Value=0.0  OutDataTypeStr=double
  Signal Specification1 : SignalSpecification  OutDataTypeStr=double  Unit=1  Dimensions=1
  Signal Specification18 : SignalSpecification  OutDataTypeStr=double  Unit=1  Dimensions=1
  Signal Specification2 : SignalSpecification  OutDataTypeStr=double  Unit=rad  Dimensions=1
  Signal Specification3 : SignalSpecification  OutDataTypeStr=double  Unit=rad  Dimensions=1
  commandedActuator : Outport
  wires:
  Signal Specification3/1 -> Bus Creator6/4  "anglePortside"
  Constant3/1 -> Signal Specification3/1
  Signal Specification2/1 -> Bus Creator6/3  "angleStarboard"
  Constant2/1 -> Signal Specification2/1
  Signal Specification1/1 -> Bus Creator6/2  "throttlePortside"
  Constant1/1 -> Signal Specification1/1
  Bus Creator6/1 -> commandedActuator/1
  Constant19/1 -> Signal Specification18/1
  Signal Specification18/1 -> Bus Creator6/1  "throttleStarboard"

== system MESSIN_Library/State Message/Empty MESSIN State Bus/Empty Control Bus ==
  Bus Creator6 : BusCreator  Inputs=2
  Constant1 : Constant  Value=false  OutDataTypeStr=boolean
  Constant19 : Constant  Value=[0;0;0]  OutDataTypeStr=double
  Signal Specification1 : SignalSpecification  OutDataTypeStr=boolean  Dimensions=1
  Signal Specification18 : SignalSpecification  OutDataTypeStr=double  Dimensions=3
  control : Outport
  wires:
  Signal Specification18/1 -> Bus Creator6/2  "XYN"
  Constant19/1 -> Signal Specification18/1
  Bus Creator6/1 -> control/1
  Constant1/1 -> Signal Specification1/1
  Signal Specification1/1 -> Bus Creator6/1  "XNAllocationEnabled"

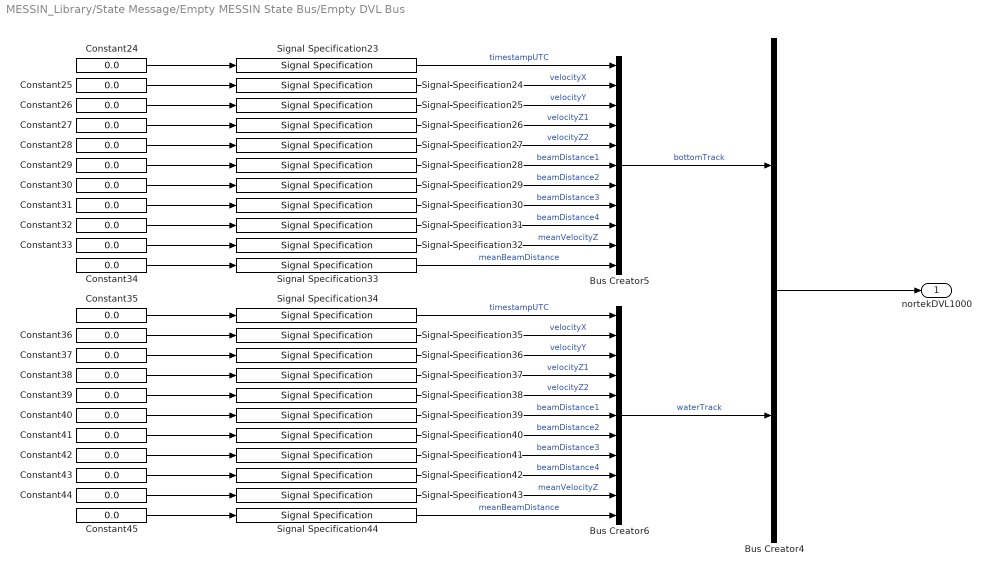
== system MESSIN_Library/State Message/Empty MESSIN State Bus/Empty DVL Bus ==
  Bus Creator4 : BusCreator  Inputs=2
  Bus Creator5 : BusCreator  Inputs=11
  Bus Creator6 : BusCreator  Inputs=11
  Constant{24..45} (22 alike) : Constant  Value=0.0  OutDataTypeStr=double
  Signal Specification23 : SignalSpecification  OutDataTypeStr=double  Unit=s  Dimensions=1
  Signal Specification{24..27,32,35..38,43} (10 alike) : SignalSpecification  OutDataTypeStr=double  Unit=m/s  Dimensions=1
  Signal Specification{28..31,33,39..42,44} (10 alike) : SignalSpecification  OutDataTypeStr=double  Unit=m  Dimensions=1
  Signal Specification34 : SignalSpecification  OutDataTypeStr=double  Unit=s  Dimensions=1
  nortekDVL1000 : Outport
  wires:
  Constant41/1 -> Signal Specification40/1
  Signal Specification41/1 -> Bus Creator6/8  "beamDistance3"
  Signal Specification28/1 -> Bus Creator5/6  "beamDistance1"
  Signal Specification33/1 -> Bus Creator5/11  "meanBeamDistance"
  Signal Specification31/1 -> Bus Creator5/9  "beamDistance4"
  Signal Specification34/1 -> Bus Creator6/1  "timestampUTC"
  Constant45/1 -> Signal Specification44/1
  Signal Specification26/1 -> Bus Creator5/4  "velocityZ1"
  Constant40/1 -> Signal Specification39/1
  Signal Specification42/1 -> Bus Creator6/9  "beamDistance4"
  Signal Specification43/1 -> Bus Creator6/10  "meanVelocityZ"
  Signal Specification32/1 -> Bus Creator5/10  "meanVelocityZ"
  Signal Specification44/1 -> Bus Creator6/11  "meanBeamDistance"
  Constant33/1 -> Signal Specification32/1
  Constant32/1 -> Signal Specification31/1
  Signal Specification38/1 -> Bus Creator6/5  "velocityZ2"
  Signal Specification27/1 -> Bus Creator5/5  "velocityZ2"
  Constant29/1 -> Signal Specification28/1
  Bus Creator4/1 -> nortekDVL1000/1
  Signal Specification30/1 -> Bus Creator5/8  "beamDistance3"
  Constant28/1 -> Signal Specification27/1
  Constant44/1 -> Signal Specification43/1
  Constant34/1 -> Signal Specification33/1
  Constant42/1 -> Signal Specification41/1
  Constant38/1 -> Signal Specification37/1
  Constant27/1 -> Signal Specification26/1
  Constant37/1 -> Signal Specification36/1
  Signal Specification23/1 -> Bus Creator5/1  "timestampUTC"
  Signal Specification39/1 -> Bus Creator6/6  "beamDistance1"
  Bus Creator6/1 -> Bus Creator4/2  "waterTrack"
  Signal Specification29/1 -> Bus Creator5/7  "beamDistance2"
  Constant31/1 -> Signal Specification30/1
  Signal Specification37/1 -> Bus Creator6/4  "velocityZ1"
  Constant39/1 -> Signal Specification38/1
  Signal Specification36/1 -> Bus Creator6/3  "velocityY"
  Constant36/1 -> Signal Specification35/1
  Constant24/1 -> Signal Specification23/1
  Constant25/1 -> Signal Specification24/1
  Constant30/1 -> Signal Specification29/1
  Constant43/1 -> Signal Specification42/1
  Signal Specification35/1 -> Bus Creator6/2  "velocityX"
  Signal Specification40/1 -> Bus Creator6/7  "beamDistance2"
  Constant35/1 -> Signal Specification34/1
  Signal Specification24/1 -> Bus Creator5/2  "velocityX"
  Bus Creator5/1 -> Bus Creator4/1  "bottomTrack"
  Signal Specification25/1 -> Bus Creator5/3  "velocityY"
  Constant26/1 -> Signal Specification25/1

== system MESSIN_Library/State Message/Empty MESSIN State Bus/Empty GNSS Bus ==
  Bus Creator3 : BusCreator  Inputs=2
  Bus Creator7 : BusCreator  Inputs=3
  Bus Creator8 : BusCreator  Inputs=7
  Constant{46,48,52..57} (8 alike) : Constant  Value=0.0  OutDataTypeStr=double
  Constant47 : Constant  Value=0  OutDataTypeStr=uint8
  Constant51 : Constant  Value=0  OutDataTypeStr=uint8
  Signal Specification45 : SignalSpecification  OutDataTypeStr=double  Unit=m  Dimensions=1
  Signal Specification46 : SignalSpecification  OutDataTypeStr=uint8  Unit=1  Dimensions=1
  Signal Specification47 : SignalSpecification  OutDataTypeStr=double  Unit=m  Dimensions=1
  Signal Specification50 : SignalSpecification  OutDataTypeStr=uint8  Unit=1  Dimensions=1
  Signal Specification51 : SignalSpecification  OutDataTypeStr=double  Unit=s  Dimensions=1
  Signal Specification52 : SignalSpecification  OutDataTypeStr=double  Unit=rad  Dimensions=1
  Signal Specification53 : SignalSpecification  OutDataTypeStr=double  Unit=m/s  Dimensions=1
  Signal Specification54 : SignalSpecification  OutDataTypeStr=double  Unit=s  Dimensions=1
  Signal Specification55 : SignalSpecification  OutDataTypeStr=double  Unit=rad  Dimensions=1
  Signal Specification56 : SignalSpecification  OutDataTypeStr=double  Unit=rad  Dimensions=1
  gnssAsteRx3 : Outport
  wires:
  Signal Specification55/1 -> Bus Creator8/2  "latitude"
  Signal Specification54/1 -> Bus Creator8/1  "timestampUTC"
  Signal Specification45/1 -> Bus Creator8/4  "altitude"
  Constant56/1 -> Signal Specification55/1
  Signal Specification46/1 -> Bus Creator8/6  "numSat"
  Signal Specification47/1 -> Bus Creator8/5  "hdop"
  Constant57/1 -> Signal Specification56/1
  Bus Creator7/1 -> Bus Creator3/2  "courseAndSpeedOverGround"
  Signal Specification52/1 -> Bus Creator7/2  "courseOverGround"
  Constant52/1 -> Signal Specification51/1
  Signal Specification56/1 -> Bus Creator8/3  "longitude"
  Signal Specification53/1 -> Bus Creator7/3  "speedOverGround"
  Constant51/1 -> Signal Specification50/1
  Constant55/1 -> Signal Specification54/1
  Constant48/1 -> Signal Specification47/1
  Signal Specification50/1 -> Bus Creator8/7  "gpsQuality"
  Bus Creator8/1 -> Bus Creator3/1  "gnss"
  Constant53/1 -> Signal Specification52/1
  Bus Creator3/1 -> gnssAsteRx3/1
  Constant54/1 -> Signal Specification53/1
  Constant46/1 -> Signal Specification45/1
  Signal Specification51/1 -> Bus Creator7/1  "timestampUTC"
  Constant47/1 -> Signal Specification46/1

== system MESSIN_Library/State Message/Empty MESSIN State Bus/Empty Guidance Bus ==
  Bus Creator : BusCreator  Inputs=2
  Bus Creator1 : BusCreator  Inputs=3
  Bus Creator6 : BusCreator  Inputs=2
  Constant{1..4,17} (5 alike) : Constant  Value=0.0  OutDataTypeStr=double
  Signal Specification1 : SignalSpecification  OutDataTypeStr=double  Unit=rad  Dimensions=1
  Signal Specification17 : SignalSpecification  OutDataTypeStr=double  Unit=m/s  Dimensions=1
  Signal Specification2 : SignalSpecification  OutDataTypeStr=double  Unit=rad  Dimensions=1
  Signal Specification3 : SignalSpecification  OutDataTypeStr=double  Unit=rad  Dimensions=1
  Signal Specification4 : SignalSpecification  OutDataTypeStr=double  Unit=m  Dimensions=1
  guidance : Outport
  wires:
  Bus Creator1/1 -> Bus Creator6/2  "stayThere"
  Constant4/1 -> Signal Specification4/1
  Constant3/1 -> Signal Specification3/1
  Constant2/1 -> Signal Specification2/1
  Signal Specification4/1 -> Bus Creator1/3  "radius"
  Signal Specification3/1 -> Bus Creator1/2  "positionLongitude"
  Signal Specification2/1 -> Bus Creator1/1  "positionLatitude"
  Bus Creator/1 -> Bus Creator6/1  "surgeHeading"
  Constant1/1 -> Signal Specification1/1
  Signal Specification1/1 -> Bus Creator/2  "orientationYaw"
  Constant17/1 -> Signal Specification17/1
  Signal Specification17/1 -> Bus Creator/1  "velocityU"
  Bus Creator6/1 -> guidance/1
